simulink model "untitled"  (R2018a)
settings: Solver=FixedStepAuto  StartTime=0.0  StopTime=10.0  FixedStep=1  RelTol=1e-3
settings Model: Creator=Ahmed-Yehia  LastModifiedBy=Ahmed-Yehia
settings OptimizationCC: DefaultParameterBehavior=Inlined  EnhancedBackFolding=on  PassReuseOutputArgsAs=Individual arguments  OptimizeBlockOrder=speed  DifferentSizesBufferReuse=on  OptimizationCustomize=off
settings DebuggingCC: UnderspecifiedInitializationDetection=Classic  MergeDetectMultiDrivingBlocksExec=none  ParameterTunabilityLossMsg=error
settings ModelReferenceCC: PropagateSignalLabelsOutOfModel=off
settings SFSimCC: MATLABDynamicMemAlloc=off
settings RTWCC: SystemTargetFile=ert.tlc  GenCodeOnly=on  TemplateMakefile=ert_default_tmf  GenerateReport=on  IncludeHyperlinkInReport=on  LaunchReport=on  GenerateTraceInfo=on  GenerateTraceReport=on  GenerateTraceReportSl=on  GenerateTraceReportSf=on  GenerateTraceReportEml=on
settings CodeAppCC: ForceParamTrailComments=on  IgnoreCustomStorageClasses=off  OperatorAnnotations=on  SimulinkDataObjDesc=on  SFDataObjDesc=on  InsertBlockDesc=on
settings ERTTargetCC: TargetLangStandard=C99 (ISO)  GenerateSampleERTMain=on  InlinedParameterPlacement=NonHierarchical  ERTCustomFileTemplate=example_file_process.tlc

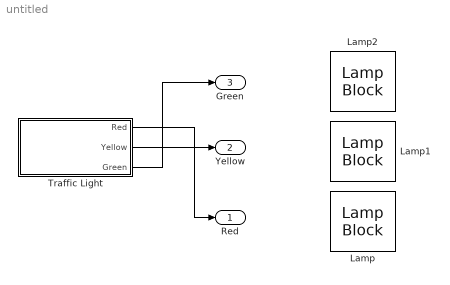
== system untitled ==
  Lamp : LampBlock  WebBlockId=2
  Lamp1 : LampBlock  WebBlockId=7
  Lamp2 : LampBlock  WebBlockId=8
  Traffic Light : Stateflow chart  TreatAsAtomicUnit=on
  Red : Outport
  Yellow : Outport  Port=2
  Green : Outport  Port=3
  wires:
  Traffic Light/3(Green) -> Green/1
  Traffic Light/1(Red) -> Red/1
  Traffic Light/2(Yellow) -> Yellow/1

== stateflow chart untitled/Traffic Light ==
  state YellowState
    en:
    Counter = 2;
    Yellow = 1;
    du:
    pause(1);
    Counter = Counter - 1;
    ex:
    Yellow = 0;
  state GreenState
    en:
    Counter = 5;
    Green = 1;
    du:
    pause(1);
    Counter = Counter - 1;
    ex:
    Green = 0;
  state RedState
    en:
    Counter = 3;
    Red = 1;
    du:
    pause(1);
    Counter = Counter - 1;
    ex:
    Red= 0;
  (default) -> GreenState
  GreenState -> YellowState : [Counter==0]
  RedState -> GreenState : [Counter==0]
  YellowState -> RedState : [Counter==0]
  data: Red output uint8; Yellow output uint8; Green output uint8; Counter local uint16
